simulink model "Cooperative_Quad_09_VelEst_02"  (R2017b)
settings: Solver=ode45  StartTime=0.0  StopTime=120  RelTol=1e-3  EnableMultiTasking=on
InitFcn:
  | Const_Vel_Est_02
values from neighbouring files (symbols this model uses):
  alpha = 1.0e-5    (= 1e-05)    [Cons_AMFC_Quad_New_01.m]    (also in Const_Vel_Est_02.m = 0.1; constant_Rev01_4Agents_10.m = 0.1; constant_Rev01_4Agents_9.m = 0.1)
  alpha_Slid = 0.01    [Cons_AMFC_Quad_New_01.m]    (also in Const_Vel_Est_02.m)
  AN = [     0 1 0 0 ... (first row only)    [Const_Vel_Est_02.m]    (also in constant_Rev01_4Agents_10.m; constant_Rev01_4Agents_9.m)
  B = 1e+0*eye(n)    [Cons_AMFC_Quad_New_01.m]    (also in Const_Vel_Est_02.m = 1e0*eye(n); constant_Rev01_4Agents_10.m = 1e0*eye(n); constant_Rev01_4Agents_9.m = 1e0*eye(n))
  BBT_inv = ((B'*B)^(-1))*B'    [Cons_AMFC_Quad_New_01.m]    (also in Const_Vel_Est_02.m; constant_Rev01_4Agents_10.m; constant_Rev01_4Agents_9.m)
  BN = [     1 0 0 0 ... (first row only)    [Const_Vel_Est_02.m]    (also in constant_Rev01_4Agents_10.m; constant_Rev01_4Agents_9.m)
  epsilon_struct = struct('data',epsilon_InitVal)    [Const_Vel_Est_02.m]    (also in constant_Rev01_4Agents_10.m; constant_Rev01_4Agents_9.m)
  g = 9.81    [Const_Vel_Est_02.m]    (also in Swing2d_01_const.m; constant_Rev01_4Agents_10.m; constant_Rev01_4Agents_9.m)
  gamma_0 = 1e-0*diag([1e-3*ones(3,1);1e-0*ones(3,1)])    [Cons_AMFC_Quad_New_01.m]    (also in Const_Vel_Est_02.m = 1e-1*diag([1e-3*ones(3,1);1e-0*ones(3,1)]); constant_Rev01_4Agents_10.m = 1e+1*diag([1e-3*ones(3,1);1e-0*ones(3,1)]); constant_Rev01_4Agents_9.m = 1e+1*diag([1e-3*ones(6,1);1e-0*ones(6,1)]))
  gamma_1 = 1e+2*diag([1e-3*ones(3,1);1e-0*ones(3,1)])    [Cons_AMFC_Quad_New_01.m]    (also in Const_Vel_Est_02.m; constant_Rev01_4Agents_10.m = 1e+3*diag([1e-3*ones(3,1);1e0*ones(3,1)]); constant_Rev01_4Agents_9.m = 1e+3*diag([1e-3*ones(6,1);1e0*ones(6,1)]))
  H = L + BN    [Const_Vel_Est_02.m]    (also in constant_Rev01_4Agents_10.m; constant_Rev01_4Agents_9.m)
  J = 1.2416e-3 * diag([1 1 2])    [Cons_AMFC_Quad_New_01.m]    (also in Const_Vel_Est_02.m = 1.2416e-3 * diag([1 1 2],0); constant_Rev01_4Agents_10.m = 1.2416e-3 * diag([1 1 2],0); constant_Rev01_4Agents_9.m = 1.2416e-3 * diag([1 1 2],0))
  k1 = 10    [Cons_AMFC_Quad_New_01.m]    (also in Const_Vel_Est_02.m = 1; constant_Rev01_4Agents_10.m = 1; constant_Rev01_4Agents_9.m = 1)
  k1o = 1000    [Cons_AMFC_Quad_New_01.m]    (also in Const_Vel_Est_02.m)
  k2 = 0.1    [Cons_AMFC_Quad_New_01.m]    (also in Const_Vel_Est_02.m; constant_Rev01_4Agents_10.m = 1; constant_Rev01_4Agents_9.m = 1)
  k2o = 100    [Cons_AMFC_Quad_New_01.m]    (also in Const_Vel_Est_02.m)
  Ka = 0.01    [Cons_AMFC_Quad_New_01.m]    (also in Const_Vel_Est_02.m; constant_Rev01_4Agents_10.m; constant_Rev01_4Agents_9.m)
  Kd = 0.01    [Cons_AMFC_Quad_New_01.m]    (also in Const_Vel_Est_02.m; constant_Rev01_4Agents_10.m; constant_Rev01_4Agents_9.m)
  Kf = 1.0e-5    (= 1e-05)    [Cons_AMFC_Quad_New_01.m]    (also in Const_Vel_Est_02.m; constant_Rev01_4Agents_10.m; constant_Rev01_4Agents_9.m)
  Kt = 0.0435 * Kf    (= 4.35e-07)    [Cons_AMFC_Quad_New_01.m]    (also in Const_Vel_Est_02.m = 1e-07; constant_Rev01_4Agents_10.m = 1e-07; constant_Rev01_4Agents_9.m = 1e-07)
  Lq = 0.2    [Const_Vel_Est_02.m]    (also in constant_Rev01_4Agents_10.m; constant_Rev01_4Agents_9.m)
  m = 6    [Cons_AMFC_Quad_New_01.m]    (also in Const_Vel_Est_02.m; Swing2d_01_const.m = 1)
  M = 2.95    [Cons_AMFC_Quad_New_01.m]    (also in Const_Vel_Est_02.m = 2; constant_Rev01_4Agents_10.m = 2; constant_Rev01_4Agents_9.m = 2)
  Mb_P = Mb_val_P*ones(np,1)    [Const_Vel_Est_02.m]
  Mb_V = Mb_val_V*ones(np,1)    [Const_Vel_Est_02.m]
  Mu_P = 10    [Const_Vel_Est_02.m]
  Mu_V = 10    [Const_Vel_Est_02.m]
  n = 6    [Cons_AMFC_Quad_New_01.m]    (also in Const_Vel_Est_02.m; constant_Rev01_4Agents_10.m; constant_Rev01_4Agents_9.m = 12)
  N = 4    [Const_Vel_Est_02.m]    (also in constant_Rev01_4Agents_10.m; constant_Rev01_4Agents_9.m)
  n0 = 3    [Const_Vel_Est_02.m]    (also in constant_Rev01_4Agents_10.m; constant_Rev01_4Agents_9.m)
  np = 2    [Const_Vel_Est_02.m]
  Observer_Gain = 100    [Const_Vel_Est_02.m]    (also in constant_Rev01_4Agents_10.m; constant_Rev01_4Agents_9.m)
  Observer_Gain1 = 100    [Const_Vel_Est_02.m]    (also in constant_Rev01_4Agents_10.m = 10; constant_Rev01_4Agents_9.m = 10)
  Q = 1e-1*eye(n)    [Cons_AMFC_Quad_New_01.m]    (also in Const_Vel_Est_02.m = 1e-2*eye(n); constant_Rev01_4Agents_10.m = 1e-3*eye(n); constant_Rev01_4Agents_9.m = 1e-3*eye(n))
  R = 1e+0*eye(m)    [Cons_AMFC_Quad_New_01.m]    (also in Const_Vel_Est_02.m = 1e-0*eye(n); constant_Rev01_4Agents_10.m = 1e-0*eye(n); constant_Rev01_4Agents_9.m = 1e-0*eye(n))
  rho_0 = 1e-1    (= 0.1)    [Cons_AMFC_Quad_New_01.m]    (also in Const_Vel_Est_02.m; constant_Rev01_4Agents_10.m = 10; constant_Rev01_4Agents_9.m = 10)
  rho_1 = 1e-0    (= 1)    [Cons_AMFC_Quad_New_01.m]    (also in Const_Vel_Est_02.m; constant_Rev01_4Agents_10.m = 0.1; constant_Rev01_4Agents_9.m = 0.1)
  T_struct = struct('data',T_InitVal)    [Const_Vel_Est_02.m]    (also in constant_Rev01_4Agents_10.m; constant_Rev01_4Agents_9.m)
  U_dot0_M = U_dot0_m*ones(n0,1)    [Const_Vel_Est_02.m]    (also in constant_Rev01_4Agents_10.m; constant_Rev01_4Agents_9.m)
  Upsilon_M = Upsilon_m*ones(n0,1)    [Const_Vel_Est_02.m]    (also in constant_Rev01_4Agents_10.m; constant_Rev01_4Agents_9.m)
undefined symbols (not defined in the file or in its folder): sigbuilder_block
(part 2 of 5)

== system Cooperative_Quad_09_VelEst_02/Agent #2/Relative estimations-2/Rel_21 ==
  A_local_XY : Inport
  P_local_XY : Inport  Port=2
  Differentiator1 : Subsystem
  Integrator1 : Integrator  InitialCondition=zeros(2,1)
  Integrator2 : Integrator  InitialCondition=zeros(2,1)
  Relative estimation1-2 : MATLAB Function  TreatAsAtomicUnit=on
  Relative estimation2 : MATLAB Function  TreatAsAtomicUnit=on
  Relative measurements2 : MATLAB Function  TreatAsAtomicUnit=on
  Sum : Sum  Inputs=|+-
  P_rel_21 : Outport
  V_rel_21 : Outport  Port=2
  wires:
  Sum/1 -> Relative estimation1-2/1(A_rel)
  [Acc1_XY] -> Sum/2
  [Pos1_XY] -> Relative measurements2/1(P_other)
  Differentiator1/1(Dx_d) -> Relative estimation1-2/2(dv)
  Relative estimation1-2/1(DV_est) -> Integrator1/1
  Relative estimation2/1(DP_est) -> Integrator2/1
  P_local_XY/1 -> Relative measurements2/2(P_local)
  A_local_XY/1 -> Sum/1
  Integrator1/1 -> Relative estimation2/1(V_rel), V_rel_21/1, Relative estimation1-2/3(V_est)
  Relative measurements2/1(d) -> Relative estimation2/2(dp), Differentiator1/1(x_d)
  Integrator2/1 -> Relative estimation2/3(P_est), P_rel_21/1

== system Cooperative_Quad_09_VelEst_02/Agent #2/Relative estimations-2/Rel_23 ==
  A_local_XY : Inport
  P_local_XY : Inport  Port=2
  Differentiator1 : Subsystem
  Integrator1 : Integrator  InitialCondition=zeros(2,1)
  Integrator2 : Integrator  InitialCondition=zeros(2,1)
  Relative estimation1-2 : MATLAB Function  TreatAsAtomicUnit=on
  Relative estimation2 : MATLAB Function  TreatAsAtomicUnit=on
  Relative measurements2 : MATLAB Function  TreatAsAtomicUnit=on
  Sum : Sum  Inputs=|+-
  P_rel_23 : Outport
  V_rel_23 : Outport  Port=2
  wires:
  Integrator2/1 -> P_rel_23/1, Relative estimation2/3(P_est)
  Relative measurements2/1(d) -> Differentiator1/1(x_d), Relative estimation2/2(dp)
  Integrator1/1 -> V_rel_23/1, Relative estimation2/1(V_rel), Relative estimation1-2/3(V_est)
  A_local_XY/1 -> Sum/1
  P_local_XY/1 -> Relative measurements2/2(P_local)
  Relative estimation2/1(DP_est) -> Integrator2/1
  Relative estimation1-2/1(DV_est) -> Integrator1/1
  Differentiator1/1(Dx_d) -> Relative estimation1-2/2(dv)
  [Pos3_XY] -> Relative measurements2/1(P_other)
  [Acc3_XY] -> Sum/2
  Sum/1 -> Relative estimation1-2/1(A_rel)

== system Cooperative_Quad_09_VelEst_02/Agent #2/Relative estimations-2/Rel_24 ==
  A_local_XY : Inport
  P_local_XY : Inport  Port=2
  Differentiator1 : Subsystem
  Integrator1 : Integrator  InitialCondition=zeros(2,1)
  Integrator2 : Integrator  InitialCondition=zeros(2,1)
  Relative estimation1 : MATLAB Function  TreatAsAtomicUnit=on
  Relative estimation2 : MATLAB Function  TreatAsAtomicUnit=on
  Relative measurements1 : MATLAB Function  TreatAsAtomicUnit=on
  Sum : Sum  Inputs=|+-
  P_rel_24 : Outport
  V_rel_24 : Outport  Port=2
  wires:
  Sum/1 -> Relative estimation2/1(A_rel)
  [Acc4_XY] -> Sum/2
  [Pos4_XY] -> Relative measurements1/1(P_other)
  Differentiator1/1(Dx_d) -> Relative estimation2/2(dv)
  Relative estimation2/1(DV_est) -> Integrator1/1
  Relative estimation1/1(DP_est) -> Integrator2/1
  P_local_XY/1 -> Relative measurements1/2(P_local)
  A_local_XY/1 -> Sum/1
  Integrator1/1 -> Relative estimation1/1(V_rel), V_rel_24/1, Relative estimation2/3(V_est)
  Relative measurements1/1(d) -> Relative estimation1/2(dp), Differentiator1/1(x_d)
  Integrator2/1 -> Relative estimation1/3(P_est), P_rel_24/1

== system Cooperative_Quad_09_VelEst_02/Agent #3/Decenteralized Cooperaive Controller #3/Ali-3 ==
  x : Inport
  xd : Inport  Port=2
  Controller interpreter-3 : MATLAB Function  TreatAsAtomicUnit=on
  Controller interpreter1-3 : MATLAB Function  TreatAsAtomicUnit=on
  Rotational-3 : Subsystem
  Translational-3 : Subsystem
  u : Outport
  wires:
  Controller interpreter-3/2(PHI_d) -> Rotational-3/1(x_rd)
  Rotational-3/1(ur) -> Controller interpreter1-3/2(ur)
  Controller interpreter1-3/1(u) -> u/1
  Controller interpreter-3/1(u0) -> Controller interpreter1-3/1(u0t)
  xd/1 -> Translational-3/1(x_td)
  x/1 -> Rotational-3/2(X), Translational-3/2(x_t)
  Translational-3/1(ut) -> Controller interpreter-3/1(u)

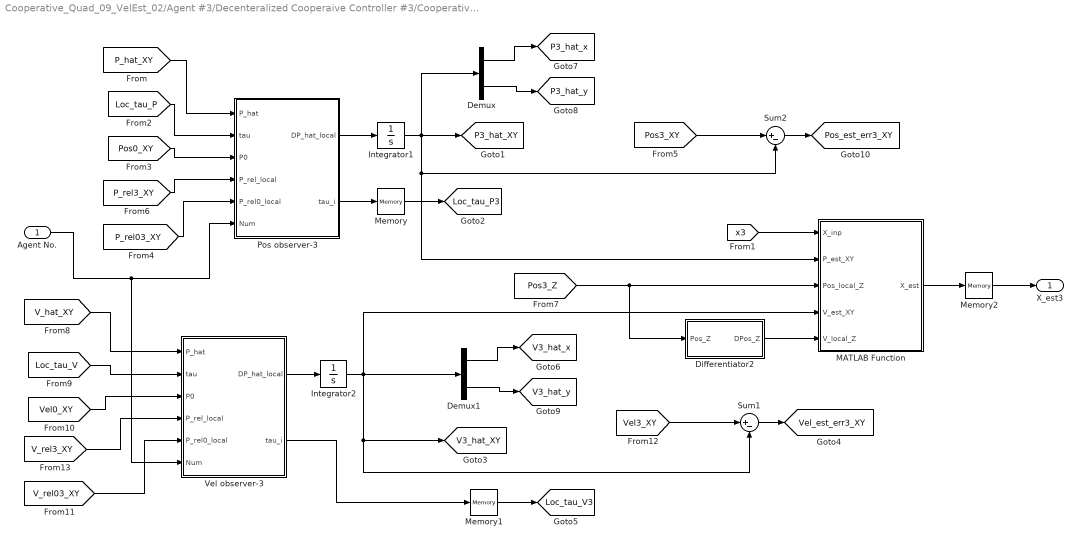
== system Cooperative_Quad_09_VelEst_02/Agent #3/Decenteralized Cooperaive Controller #3/Cooperative Observers for X-3 ==
  Agent No. : Inport
  Demux : Demux  Outputs=2
  Demux1 : Demux  Outputs=2
  Differentiator2 : Subsystem
  Integrator1 : Integrator  InitialCondition=zeros(np,1)
  Integrator2 : Integrator  InitialCondition=zeros(np,1)
  MATLAB Function : MATLAB Function  TreatAsAtomicUnit=on
  Memory : Memory  InitialCondition=zeros(np,1)
  Memory1 : Memory  InitialCondition=zeros(np,1)
  Memory2 : Memory  InitialCondition=zeros(2*n,1)
  Pos observer-3 : MATLAB Function  TreatAsAtomicUnit=on
  Sum1 : Sum  Inputs=|+-
  Sum2 : Sum  Inputs=|+-
  Vel observer-3 : MATLAB Function  TreatAsAtomicUnit=on
  X_est3 : Outport
  tag scope: Loc_tau_P3=global, Loc_tau_V3=global, P3_hat_XY=global, P3_hat_x=global, P3_hat_y=global, Pos_est_err3_XY=global, V3_hat_XY=global, V3_hat_x=global, V3_hat_y=global, Vel_est_err3_XY=global
  wires:
  [Pos3_XY] -> Sum2/1
  [Loc_tau_P] -> Pos observer-3/2(tau)
  [P_rel03_XY] -> Pos observer-3/5(P_rel0_local)
  Pos observer-3/1(DP_hat_local) -> Integrator1/1
  Pos observer-3/2(tau_i) -> Memory/1
  Demux/1 -> [P3_hat_x]
  Memory/1 -> [Loc_tau_P3]
  [Pos0_XY] -> Pos observer-3/3(P0)
  [P_hat_XY] -> Pos observer-3/1(P_hat)
  Sum2/1 -> [Pos_est_err3_XY]
  [P_rel3_XY] -> Pos observer-3/4(P_rel_local)
  Demux/2 -> [P3_hat_y]
  Integrator1/1 -> Sum2/2, MATLAB Function/2(P_est_XY), Demux/1, [P3_hat_XY]
  Agent No./1 -> Vel observer-3/6(Num), Pos observer-3/6(Num)
  MATLAB Function/1(X_est) -> Memory2/1
  [x3] -> MATLAB Function/1(X_inp)
  [Pos3_Z] -> Differentiator2/1(Pos_Z), MATLAB Function/3(Pos_local_Z)
  Differentiator2/1(DPos_Z) -> MATLAB Function/5(V_local_Z)
  [Vel3_XY] -> Sum1/1
  Integrator2/1 -> Sum1/2, [V3_hat_XY], Demux1/1, MATLAB Function/4(V_est_XY)
  Demux1/2 -> [V3_hat_y]
  [V_rel3_XY] -> Vel observer-3/4(P_rel_local)
  [Loc_tau_V] -> Vel observer-3/2(tau)
  [V_hat_XY] -> Vel observer-3/1(P_hat)
  Sum1/1 -> [Vel_est_err3_XY]
  [V_rel03_XY] -> Vel observer-3/5(P_rel0_local)
  [Vel0_XY] -> Vel observer-3/3(P0)
  Demux1/1 -> [V3_hat_x]
  Memory1/1 -> [Loc_tau_V3]
  Vel observer-3/2(tau_i) -> Memory1/1
  Vel observer-3/1(DP_hat_local) -> Integrator2/1
  Memory2/1 -> X_est3/1

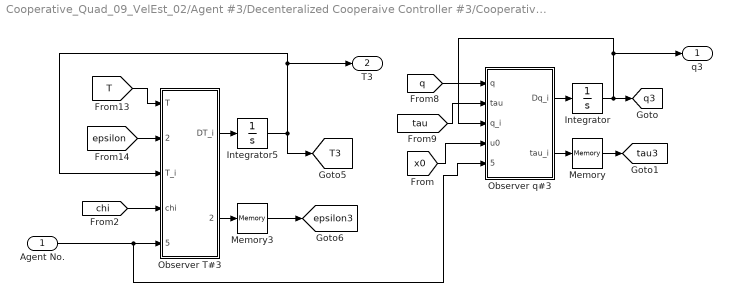
== system Cooperative_Quad_09_VelEst_02/Agent #3/Decenteralized Cooperaive Controller #3/Cooperative Observers for Xd-3 ==
  Agent No. : Inport
  Integrator : Integrator  InitialCondition=zeros(n0,1)
  Integrator5 : Integrator  InitialCondition=zeros(N+1,n0)
  Memory : Memory  InitialCondition=zeros(n0,1)
  Memory3 : Memory  InitialCondition=zeros(N+1,n0)
  Observer T#3 : MATLAB Function  TreatAsAtomicUnit=on
  Observer q#3 : MATLAB Function  TreatAsAtomicUnit=on
  q3 : Outport
  T3 : Outport  Port=2
  tag scope: T3=global, epsilon3=global, q3=global, tau3=global
  wires:
  [chi] -> Observer T#3/4(chi)
  [epsilon] -> Observer T#3/2(epsilon)
  Observer T#3/1(DT_i) -> Integrator5/1
  [T] -> Observer T#3/1(T)
  Observer T#3/2(epsilon_i) -> Memory3/1
  Observer q#3/1(Dq_i) -> Integrator/1
  Memory/1 -> [tau3]
  [x0] -> Observer q#3/4(u0)
  Observer q#3/2(tau_i) -> Memory/1
  Agent No./1 -> Observer q#3/5(Agent_Num), Observer T#3/5(Agent_Num)
  Integrator5/1 -> [T3], T3/1, Observer T#3/3(T_i)
  [q] -> Observer q#3/1(q)
  Integrator/1 -> [q3], q3/1, Observer q#3/3(q_i)
  [tau] -> Observer q#3/2(tau)
  Memory3/1 -> [epsilon3]

== system Cooperative_Quad_09_VelEst_02/Agent #3/Decenteralized Cooperaive Controller #3/Subsystem ==
  In1 : Inport
  Demux : Demux  Outputs=3
  Mux : Mux  Inputs=3
  Transport Delay1 : TransportDelay  DelayTime=5
  Transport Delay2 : TransportDelay  DelayTime=5
  Out1 : Outport
  wires:
  In1/1 -> Demux/1
  Demux/1 -> Transport Delay1/1
  Demux/2 -> Transport Delay2/1
  Mux/1 -> Out1/1
  Transport Delay2/1 -> Mux/2
  Transport Delay1/1 -> Mux/1
  Demux/3 -> Mux/3

== system Cooperative_Quad_09_VelEst_02/Agent #3/Relative estimations-3/Rel_30 ==
  A_local_XY : Inport
  P_local_XY : Inport  Port=2
  Differentiator1 : Subsystem
  Integrator1 : Integrator  InitialCondition=zeros(2,1)
  Integrator2 : Integrator  InitialCondition=zeros(2,1)
  Relative estimation1 : MATLAB Function  TreatAsAtomicUnit=on
  Relative estimation2 : MATLAB Function  TreatAsAtomicUnit=on
  Relative measurements1 : MATLAB Function  TreatAsAtomicUnit=on
  Sum : Sum  Inputs=|+-
  P_rel_30 : Outport
  V_rel_30 : Outport  Port=2
  wires:
  Sum/1 -> Relative estimation2/1(A_rel)
  [Acc0_XY] -> Sum/2
  [Pos0_XY] -> Relative measurements1/1(P_other)
  Differentiator1/1(Dx_d) -> Relative estimation2/2(dv)
  Relative estimation2/1(DV_est) -> Integrator1/1
  Relative estimation1/1(DP_est) -> Integrator2/1
  P_local_XY/1 -> Relative measurements1/2(P_local)
  A_local_XY/1 -> Sum/1
  Integrator1/1 -> Relative estimation1/1(V_rel), V_rel_30/1, Relative estimation2/3(V_est)
  Relative measurements1/1(d) -> Relative estimation1/2(dp), Differentiator1/1(x_d)
  Integrator2/1 -> Relative estimation1/3(P_est), P_rel_30/1

== system Cooperative_Quad_09_VelEst_02/Agent #3/Relative estimations-3/Rel_31 ==
  A_local_XY : Inport
  P_local_XY : Inport  Port=2
  Differentiator1 : Subsystem
  Integrator1 : Integrator  InitialCondition=zeros(2,1)
  Integrator2 : Integrator  InitialCondition=zeros(2,1)
  Relative estimation1-2 : MATLAB Function  TreatAsAtomicUnit=on
  Relative estimation2 : MATLAB Function  TreatAsAtomicUnit=on
  Relative measurements2 : MATLAB Function  TreatAsAtomicUnit=on
  Sum : Sum  Inputs=|+-
  P_rel_31 : Outport
  V_rel_31 : Outport  Port=2
  wires:
  Integrator2/1 -> P_rel_31/1, Relative estimation2/3(P_est)
  Relative measurements2/1(d) -> Differentiator1/1(x_d), Relative estimation2/2(dp)
  Integrator1/1 -> Relative estimation1-2/3(V_est), V_rel_31/1, Relative estimation2/1(V_rel)
  A_local_XY/1 -> Sum/1
  P_local_XY/1 -> Relative measurements2/2(P_local)
  Relative estimation2/1(DP_est) -> Integrator2/1
  Relative estimation1-2/1(DV_est) -> Integrator1/1
  Differentiator1/1(Dx_d) -> Relative estimation1-2/2(dv)
  [Pos1_XY] -> Relative measurements2/1(P_other)
  [Acc1_XY] -> Sum/2
  Sum/1 -> Relative estimation1-2/1(A_rel)

== system Cooperative_Quad_09_VelEst_02/Agent #3/Relative estimations-3/Rel_32 ==
  A_local_XY : Inport
  P_local_XY : Inport  Port=2
  Differentiator1 : Subsystem
  Integrator1 : Integrator  InitialCondition=zeros(2,1)
  Integrator2 : Integrator  InitialCondition=zeros(2,1)
  Relative estimation1-2 : MATLAB Function  TreatAsAtomicUnit=on
  Relative estimation2 : MATLAB Function  TreatAsAtomicUnit=on
  Relative measurements2 : MATLAB Function  TreatAsAtomicUnit=on
  Sum : Sum  Inputs=|+-
  P_rel_32 : Outport
  V_rel_32 : Outport  Port=2
  wires:
  Sum/1 -> Relative estimation1-2/1(A_rel)
  [Acc2_XY] -> Sum/2
  [Pos2_XY] -> Relative measurements2/1(P_other)
  Differentiator1/1(Dx_d) -> Relative estimation1-2/2(dv)
  Relative estimation1-2/1(DV_est) -> Integrator1/1
  Relative estimation2/1(DP_est) -> Integrator2/1
  P_local_XY/1 -> Relative measurements2/2(P_local)
  A_local_XY/1 -> Sum/1
  Integrator1/1 -> Relative estimation1-2/3(V_est), Relative estimation2/1(V_rel), V_rel_32/1
  Relative measurements2/1(d) -> Relative estimation2/2(dp), Differentiator1/1(x_d)
  Integrator2/1 -> Relative estimation2/3(P_est), P_rel_32/1

== system Cooperative_Quad_09_VelEst_02/Agent #3/Relative estimations-3/Rel_34 ==
  A_local_XY : Inport
  P_local_XY : Inport  Port=2
  Differentiator1 : Subsystem
  Integrator1 : Integrator  InitialCondition=zeros(2,1)
  Integrator2 : Integrator  InitialCondition=zeros(2,1)
  Relative estimation1 : MATLAB Function  TreatAsAtomicUnit=on
  Relative estimation2 : MATLAB Function  TreatAsAtomicUnit=on
  Relative measurements1 : MATLAB Function  TreatAsAtomicUnit=on
  Sum : Sum  Inputs=|+-
  P_rel_34 : Outport
  V_rel_34 : Outport  Port=2
  wires:
  Integrator2/1 -> P_rel_34/1, Relative estimation1/3(P_est)
  Relative measurements1/1(d) -> Differentiator1/1(x_d), Relative estimation1/2(dp)
  Integrator1/1 -> Relative estimation2/3(V_est), V_rel_34/1, Relative estimation1/1(V_rel)
  A_local_XY/1 -> Sum/1
  P_local_XY/1 -> Relative measurements1/2(P_local)
  Relative estimation1/1(DP_est) -> Integrator2/1
  Relative estimation2/1(DV_est) -> Integrator1/1
  Differentiator1/1(Dx_d) -> Relative estimation2/2(dv)
  [Pos4_XY] -> Relative measurements1/1(P_other)
  [Acc4_XY] -> Sum/2
  Sum/1 -> Relative estimation2/1(A_rel)

== system Cooperative_Quad_09_VelEst_02/Agent #4/Decenteralized Cooperaive Controller #4/Ali-4 ==
  x : Inport
  xd : Inport  Port=2
  Controller interpreter-4 : MATLAB Function  TreatAsAtomicUnit=on
  Controller interpreter1-4 : MATLAB Function  TreatAsAtomicUnit=on
  Rotational-4 : Subsystem
  Translational-4 : Subsystem
  u : Outport
  wires:
  Translational-4/1(ut) -> Controller interpreter-4/1(u)
  x/1 -> Translational-4/2(x_t), Rotational-4/2(X)
  xd/1 -> Translational-4/1(x_td)
  Controller interpreter-4/1(u0) -> Controller interpreter1-4/1(u0t)
  Controller interpreter1-4/1(u) -> u/1
  Rotational-4/1(ur) -> Controller interpreter1-4/2(ur)
  Controller interpreter-4/2(PHI_d) -> Rotational-4/1(x_rd)

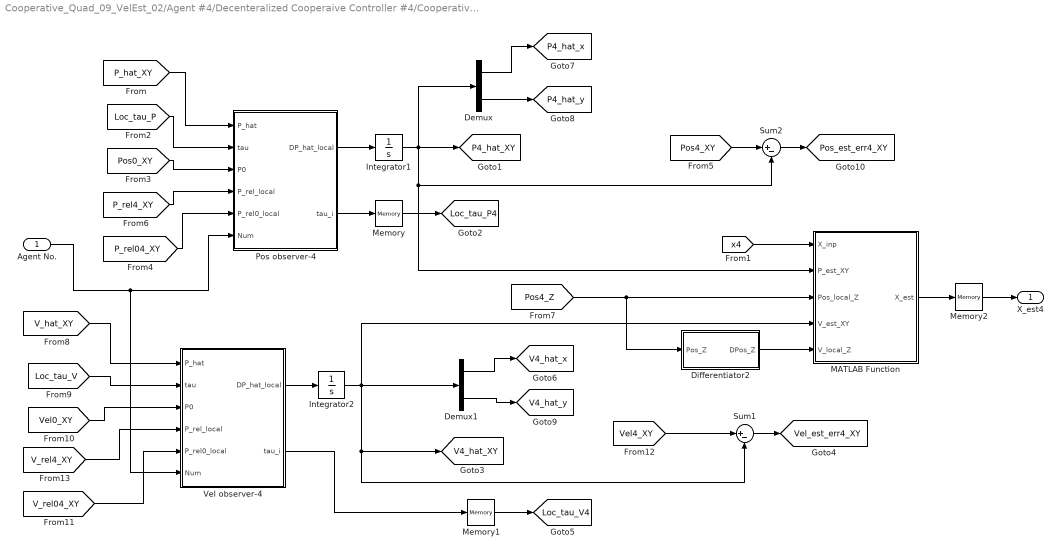
== system Cooperative_Quad_09_VelEst_02/Agent #4/Decenteralized Cooperaive Controller #4/Cooperative Observers for X-4 ==
  Agent No. : Inport
  Demux : Demux  Outputs=2
  Demux1 : Demux  Outputs=2
  Differentiator2 : Subsystem
  Integrator1 : Integrator  InitialCondition=zeros(np,1)
  Integrator2 : Integrator  InitialCondition=zeros(np,1)
  MATLAB Function : MATLAB Function  TreatAsAtomicUnit=on
  Memory : Memory  InitialCondition=zeros(np,1)
  Memory1 : Memory  InitialCondition=zeros(np,1)
  Memory2 : Memory  InitialCondition=zeros(2*n,1)
  Pos observer-4 : MATLAB Function  TreatAsAtomicUnit=on
  Sum1 : Sum  Inputs=|+-
  Sum2 : Sum  Inputs=|+-
  Vel observer-4 : MATLAB Function  TreatAsAtomicUnit=on
  X_est4 : Outport
  tag scope: Loc_tau_P4=global, Loc_tau_V4=global, P4_hat_XY=global, P4_hat_x=global, P4_hat_y=global, Pos_est_err4_XY=global, V4_hat_XY=global, V4_hat_x=global, V4_hat_y=global, Vel_est_err4_XY=global
  wires:
  Vel observer-4/1(DP_hat_local) -> Integrator2/1
  Vel observer-4/2(tau_i) -> Memory1/1
  Memory1/1 -> [Loc_tau_V4]
  Demux1/1 -> [V4_hat_x]
  [Vel0_XY] -> Vel observer-4/3(P0)
  [V_rel04_XY] -> Vel observer-4/5(P_rel0_local)
  Sum1/1 -> [Vel_est_err4_XY]
  [V_hat_XY] -> Vel observer-4/1(P_hat)
  [Loc_tau_V] -> Vel observer-4/2(tau)
  [V_rel4_XY] -> Vel observer-4/4(P_rel_local)
  Demux1/2 -> [V4_hat_y]
  Integrator2/1 -> MATLAB Function/4(V_est_XY), Demux1/1, [V4_hat_XY], Sum1/2
  [Vel4_XY] -> Sum1/1
  Differentiator2/1(DPos_Z) -> MATLAB Function/5(V_local_Z)
  [Pos4_Z] -> MATLAB Function/3(Pos_local_Z), Differentiator2/1(Pos_Z)
  [x4] -> MATLAB Function/1(X_inp)
  MATLAB Function/1(X_est) -> Memory2/1
  Agent No./1 -> Pos observer-4/6(Num), Vel observer-4/6(Num)
  Integrator1/1 -> [P4_hat_XY], Demux/1, MATLAB Function/2(P_est_XY), Sum2/2
  Demux/2 -> [P4_hat_y]
  [P_rel4_XY] -> Pos observer-4/4(P_rel_local)
  Sum2/1 -> [Pos_est_err4_XY]
  [P_hat_XY] -> Pos observer-4/1(P_hat)
  [Pos0_XY] -> Pos observer-4/3(P0)
  Memory/1 -> [Loc_tau_P4]
  Demux/1 -> [P4_hat_x]
  Pos observer-4/2(tau_i) -> Memory/1
  Pos observer-4/1(DP_hat_local) -> Integrator1/1
  [P_rel04_XY] -> Pos observer-4/5(P_rel0_local)
  [Loc_tau_P] -> Pos observer-4/2(tau)
  [Pos4_XY] -> Sum2/1
  Memory2/1 -> X_est4/1

== system Cooperative_Quad_09_VelEst_02/Agent #4/Decenteralized Cooperaive Controller #4/Cooperative Observers for Xd-4 ==
  Agent No. : Inport
  Integrator : Integrator  InitialCondition=zeros(n0,1)
  Integrator5 : Integrator  InitialCondition=zeros(N+1,n0)
  Memory : Memory  InitialCondition=zeros(n0,1)
  Memory3 : Memory  InitialCondition=zeros(N+1,n0)
  Observer T#4 : MATLAB Function  TreatAsAtomicUnit=on
  Observer q#4 : MATLAB Function  TreatAsAtomicUnit=on
  q4 : Outport
  T4 : Outport  Port=2
  tag scope: T4=global, epsilon4=global, q4=global, tau4=global
  wires:
  Memory3/1 -> [epsilon4]
  [tau] -> Observer q#4/2(tau)
  Integrator/1 -> Observer q#4/3(q_i), q4/1, [q4]
  [q] -> Observer q#4/1(q)
  Integrator5/1 -> Observer T#4/3(T_i), T4/1, [T4]
  Agent No./1 -> Observer T#4/5(Agent_Num), Observer q#4/5(Agent_Num)
  Observer q#4/2(tau_i) -> Memory/1
  [x0] -> Observer q#4/4(u0)
  Memory/1 -> [tau4]
  Observer q#4/1(Dq_i) -> Integrator/1
  Observer T#4/2(epsilon_i) -> Memory3/1
  [T] -> Observer T#4/1(T)
  Observer T#4/1(DT_i) -> Integrator5/1
  [epsilon] -> Observer T#4/2(epsilon)
  [chi] -> Observer T#4/4(chi)

== system Cooperative_Quad_09_VelEst_02/Agent #4/Decenteralized Cooperaive Controller #4/Subsystem ==
  In1 : Inport
  Demux : Demux  Outputs=3
  Mux : Mux  Inputs=3
  Transport Delay1 : TransportDelay  DelayTime=5
  Transport Delay2 : TransportDelay  DelayTime=5
  Out1 : Outport
  wires:
  Demux/3 -> Mux/3
  Transport Delay1/1 -> Mux/1
  Transport Delay2/1 -> Mux/2
  Mux/1 -> Out1/1
  Demux/2 -> Transport Delay2/1
  Demux/1 -> Transport Delay1/1
  In1/1 -> Demux/1

== system Cooperative_Quad_09_VelEst_02/Agent #4/Relative estimations-4/Rel_40 ==
  A_local_XY : Inport
  P_local_XY : Inport  Port=2
  Differentiator1 : Subsystem
  Integrator1 : Integrator  InitialCondition=zeros(2,1)
  Integrator2 : Integrator  InitialCondition=zeros(2,1)
  Relative estimation1 : MATLAB Function  TreatAsAtomicUnit=on
  Relative estimation2 : MATLAB Function  TreatAsAtomicUnit=on
  Relative measurements1 : MATLAB Function  TreatAsAtomicUnit=on
  Sum : Sum  Inputs=|+-
  P_rel_40 : Outport
  V_rel_40 : Outport  Port=2
  wires:
  Integrator2/1 -> P_rel_40/1, Relative estimation1/3(P_est)
  Relative measurements1/1(d) -> Differentiator1/1(x_d), Relative estimation1/2(dp)
  Integrator1/1 -> Relative estimation2/3(V_est), V_rel_40/1, Relative estimation1/1(V_rel)
  A_local_XY/1 -> Sum/1
  P_local_XY/1 -> Relative measurements1/2(P_local)
  Relative estimation1/1(DP_est) -> Integrator2/1
  Relative estimation2/1(DV_est) -> Integrator1/1
  Differentiator1/1(Dx_d) -> Relative estimation2/2(dv)
  [Pos0_XY] -> Relative measurements1/1(P_other)
  [Acc0_XY] -> Sum/2
  Sum/1 -> Relative estimation2/1(A_rel)

== system Cooperative_Quad_09_VelEst_02/Agent #4/Relative estimations-4/Rel_41 ==
  A_local_XY : Inport
  P_local_XY : Inport  Port=2
  Differentiator1 : Subsystem
  Integrator1 : Integrator  InitialCondition=zeros(2,1)
  Integrator2 : Integrator  InitialCondition=zeros(2,1)
  Relative estimation1-2 : MATLAB Function  TreatAsAtomicUnit=on
  Relative estimation2 : MATLAB Function  TreatAsAtomicUnit=on
  Relative measurements2 : MATLAB Function  TreatAsAtomicUnit=on
  Sum : Sum  Inputs=|+-
  P_rel_41 : Outport
  V_rel_41 : Outport  Port=2
  wires:
  Sum/1 -> Relative estimation1-2/1(A_rel)
  [Acc1_XY] -> Sum/2
  [Pos1_XY] -> Relative measurements2/1(P_other)
  Differentiator1/1(Dx_d) -> Relative estimation1-2/2(dv)
  Relative estimation1-2/1(DV_est) -> Integrator1/1
  Relative estimation2/1(DP_est) -> Integrator2/1
  P_local_XY/1 -> Relative measurements2/2(P_local)
  A_local_XY/1 -> Sum/1
  Integrator1/1 -> Relative estimation2/1(V_rel), V_rel_41/1, Relative estimation1-2/3(V_est)
  Relative measurements2/1(d) -> Relative estimation2/2(dp), Differentiator1/1(x_d)
  Integrator2/1 -> Relative estimation2/3(P_est), P_rel_41/1

== system Cooperative_Quad_09_VelEst_02/Agent #4/Relative estimations-4/Rel_42 ==
  A_local_XY : Inport
  P_local_XY : Inport  Port=2
  Differentiator1 : Subsystem
  Integrator1 : Integrator  InitialCondition=zeros(2,1)
  Integrator2 : Integrator  InitialCondition=zeros(2,1)
  Relative estimation1-2 : MATLAB Function  TreatAsAtomicUnit=on
  Relative estimation2 : MATLAB Function  TreatAsAtomicUnit=on
  Relative measurements2 : MATLAB Function  TreatAsAtomicUnit=on
  Sum : Sum  Inputs=|+-
  P_rel_42 : Outport
  V_rel_42 : Outport  Port=2
  wires:
  Integrator2/1 -> P_rel_42/1, Relative estimation2/3(P_est)
  Relative measurements2/1(d) -> Differentiator1/1(x_d), Relative estimation2/2(dp)
  Integrator1/1 -> V_rel_42/1, Relative estimation2/1(V_rel), Relative estimation1-2/3(V_est)
  A_local_XY/1 -> Sum/1
  P_local_XY/1 -> Relative measurements2/2(P_local)
  Relative estimation2/1(DP_est) -> Integrator2/1
  Relative estimation1-2/1(DV_est) -> Integrator1/1
  Differentiator1/1(Dx_d) -> Relative estimation1-2/2(dv)
  [Pos2_XY] -> Relative measurements2/1(P_other)
  [Acc2_XY] -> Sum/2
  Sum/1 -> Relative estimation1-2/1(A_rel)

== system Cooperative_Quad_09_VelEst_02/Agent #4/Relative estimations-4/Rel_43 ==
  A_local_XY : Inport
  P_local_XY : Inport  Port=2
  Differentiator1 : Subsystem
  Integrator1 : Integrator  InitialCondition=zeros(2,1)
  Integrator2 : Integrator  InitialCondition=zeros(2,1)
  Relative estimation1 : MATLAB Function  TreatAsAtomicUnit=on
  Relative estimation2 : MATLAB Function  TreatAsAtomicUnit=on
  Relative measurements1 : MATLAB Function  TreatAsAtomicUnit=on
  Sum : Sum  Inputs=|+-
  P_rel_43 : Outport
  V_rel_43 : Outport  Port=2
  wires:
  Sum/1 -> Relative estimation2/1(A_rel)
  [Acc3_XY] -> Sum/2
  [Pos3_XY] -> Relative measurements1/1(P_other)
  Differentiator1/1(Dx_d) -> Relative estimation2/2(dv)
  Relative estimation2/1(DV_est) -> Integrator1/1
  Relative estimation1/1(DP_est) -> Integrator2/1
  P_local_XY/1 -> Relative measurements1/2(P_local)
  A_local_XY/1 -> Sum/1
  Integrator1/1 -> Relative estimation1/1(V_rel), V_rel_43/1, Relative estimation2/3(V_est)
  Relative measurements1/1(d) -> Relative estimation1/2(dp), Differentiator1/1(x_d)
  Integrator2/1 -> Relative estimation1/3(P_est), P_rel_43/1

== system Cooperative_Quad_09_VelEst_02/Data Bus /Communications for controllers/For matrix Plot ==
  P : Inport
  MATLAB Function : MATLAB Function  TreatAsAtomicUnit=on
  Scope24 : Scope
  To Workspace : ToWorkspace  VariableName=P1_T  SaveFormat=Structure With Time  SampleTime=-1
  wires:
  P/1 -> MATLAB Function/1(u)
  MATLAB Function/1(y) -> Scope24/1, To Workspace/1

== system Cooperative_Quad_09_VelEst_02/Data Bus /Communications for controllers/For matrix Plot1 ==
  P : Inport
  MATLAB Function : MATLAB Function  TreatAsAtomicUnit=on
  Scope24 : Scope
  To Workspace : ToWorkspace  VariableName=P2_T  SaveFormat=Structure With Time  SampleTime=-1
  wires:
  MATLAB Function/1(y) -> Scope24/1, To Workspace/1
  P/1 -> MATLAB Function/1(u)

== system Cooperative_Quad_09_VelEst_02/Data Bus /Communications for controllers/For matrix Plot16 ==
  P : Inport
  MATLAB Function : MATLAB Function  TreatAsAtomicUnit=on
  Scope24 : Scope
  To Workspace : ToWorkspace  VariableName=P1_R  SaveFormat=Structure With Time  SampleTime=-1
  wires:
  MATLAB Function/1(y) -> To Workspace/1, Scope24/1
  P/1 -> MATLAB Function/1(u)

== system Cooperative_Quad_09_VelEst_02/Data Bus /Communications for controllers/For matrix Plot17 ==
  P : Inport
  MATLAB Function : MATLAB Function  TreatAsAtomicUnit=on
  Scope24 : Scope
  To Workspace : ToWorkspace  VariableName=P2_R  SaveFormat=Structure With Time  SampleTime=-1
  wires:
  P/1 -> MATLAB Function/1(u)
  MATLAB Function/1(y) -> To Workspace/1, Scope24/1

== system Cooperative_Quad_09_VelEst_02/Data Bus /Communications for controllers/For matrix Plot18 ==
  P : Inport
  MATLAB Function : MATLAB Function  TreatAsAtomicUnit=on
  Scope24 : Scope
  To Workspace : ToWorkspace  VariableName=P3_R  SaveFormat=Structure With Time  SampleTime=-1
  wires:
  P/1 -> MATLAB Function/1(u)
  MATLAB Function/1(y) -> To Workspace/1, Scope24/1

== system Cooperative_Quad_09_VelEst_02/Data Bus /Communications for controllers/For matrix Plot19 ==
  P : Inport
  MATLAB Function : MATLAB Function  TreatAsAtomicUnit=on
  Scope24 : Scope
  To Workspace : ToWorkspace  VariableName=P4_R  SaveFormat=Structure With Time  SampleTime=-1
  wires:
  MATLAB Function/1(y) -> To Workspace/1, Scope24/1
  P/1 -> MATLAB Function/1(u)

== system Cooperative_Quad_09_VelEst_02/Data Bus /Communications for controllers/For matrix Plot2 ==
  P : Inport
  MATLAB Function : MATLAB Function  TreatAsAtomicUnit=on
  Scope24 : Scope
  To Workspace : ToWorkspace  VariableName=P3_T  SaveFormat=Structure With Time  SampleTime=-1
  wires:
  MATLAB Function/1(y) -> Scope24/1, To Workspace/1
  P/1 -> MATLAB Function/1(u)

== system Cooperative_Quad_09_VelEst_02/Data Bus /Communications for controllers/For matrix Plot20 ==
  A_hat : Inport
  MATLAB Function : MATLAB Function  TreatAsAtomicUnit=on
  Scope24 : Scope
  To Workspace : ToWorkspace  VariableName=A_hat1_R  SaveFormat=Structure With Time  SampleTime=-1
  wires:
  A_hat/1 -> MATLAB Function/1(u)
  MATLAB Function/1(y) -> To Workspace/1, Scope24/1

== system Cooperative_Quad_09_VelEst_02/Data Bus /Communications for controllers/For matrix Plot21 ==
  A_hat : Inport
  MATLAB Function : MATLAB Function  TreatAsAtomicUnit=on
  Scope24 : Scope
  To Workspace : ToWorkspace  VariableName=A_hat2_R  SaveFormat=Structure With Time  SampleTime=-1
  wires:
  MATLAB Function/1(y) -> To Workspace/1, Scope24/1
  A_hat/1 -> MATLAB Function/1(u)

== system Cooperative_Quad_09_VelEst_02/Data Bus /Communications for controllers/For matrix Plot22 ==
  A_hat : Inport
  MATLAB Function : MATLAB Function  TreatAsAtomicUnit=on
  Scope24 : Scope
  To Workspace : ToWorkspace  VariableName=A_hat3_R  SaveFormat=Structure With Time  SampleTime=-1
  wires:
  A_hat/1 -> MATLAB Function/1(u)
  MATLAB Function/1(y) -> To Workspace/1, Scope24/1

== system Cooperative_Quad_09_VelEst_02/Data Bus /Communications for controllers/For matrix Plot23 ==
  A_hat : Inport
  MATLAB Function : MATLAB Function  TreatAsAtomicUnit=on
  Scope24 : Scope
  To Workspace : ToWorkspace  VariableName=A_hat4_R  SaveFormat=Structure With Time  SampleTime=-1
  wires:
  MATLAB Function/1(y) -> To Workspace/1, Scope24/1
  A_hat/1 -> MATLAB Function/1(u)

== system Cooperative_Quad_09_VelEst_02/Data Bus /Communications for controllers/For matrix Plot3 ==
  P : Inport
  MATLAB Function : MATLAB Function  TreatAsAtomicUnit=on
  Scope24 : Scope
  To Workspace : ToWorkspace  VariableName=P4_T  SaveFormat=Structure With Time  SampleTime=-1
  wires:
  P/1 -> MATLAB Function/1(u)
  MATLAB Function/1(y) -> Scope24/1, To Workspace/1

== system Cooperative_Quad_09_VelEst_02/Data Bus /Communications for controllers/For matrix Plot4 ==
  A_hat : Inport
  MATLAB Function : MATLAB Function  TreatAsAtomicUnit=on
  Scope24 : Scope
  To Workspace : ToWorkspace  VariableName=A_hat1_T  SaveFormat=Structure With Time  SampleTime=-1
  wires:
  MATLAB Function/1(y) -> Scope24/1, To Workspace/1
  A_hat/1 -> MATLAB Function/1(u)

== system Cooperative_Quad_09_VelEst_02/Data Bus /Communications for controllers/For matrix Plot5 ==
  A_hat : Inport
  MATLAB Function : MATLAB Function  TreatAsAtomicUnit=on
  Scope24 : Scope
  To Workspace : ToWorkspace  VariableName=A_hat2_T  SaveFormat=Structure With Time  SampleTime=-1
  wires:
  A_hat/1 -> MATLAB Function/1(u)
  MATLAB Function/1(y) -> Scope24/1, To Workspace/1

== system Cooperative_Quad_09_VelEst_02/Data Bus /Communications for controllers/For matrix Plot6 ==
  A_hat : Inport
  MATLAB Function : MATLAB Function  TreatAsAtomicUnit=on
  Scope24 : Scope
  To Workspace : ToWorkspace  VariableName=A_hat3_T  SaveFormat=Structure With Time  SampleTime=-1
  wires:
  MATLAB Function/1(y) -> Scope24/1, To Workspace/1
  A_hat/1 -> MATLAB Function/1(u)

== system Cooperative_Quad_09_VelEst_02/Data Bus /Communications for controllers/For matrix Plot7 ==
  A_hat : Inport
  MATLAB Function : MATLAB Function  TreatAsAtomicUnit=on
  Scope24 : Scope
  To Workspace : ToWorkspace  VariableName=A_hat4_T  SaveFormat=Structure With Time  SampleTime=-1
  wires:
  A_hat/1 -> MATLAB Function/1(u)
  MATLAB Function/1(y) -> Scope24/1, To Workspace/1

== system Cooperative_Quad_09_VelEst_02/Data Bus /Reference Trajectory/Differentiator ==
  x_d : Inport
  Integrator : Integrator  InitialCondition=zeros(np,1)
  Integrator1 : Integrator  InitialCondition=zeros(np,1)
  Sliding differentiator : MATLAB Function  TreatAsAtomicUnit=on
  Sliding differentiator1 : MATLAB Function  TreatAsAtomicUnit=on
  Sum : Sum  Inputs=|-+
  Dx_d : Outport
  wires:
  Integrator1/1 -> Sum/2
  Sum/1 -> Sliding differentiator1/1(e), Sliding differentiator/2(e)
  x_d/1 -> Sum/1
  Integrator/1 -> Sliding differentiator/1(u1)
  Sliding differentiator1/1(Du1) -> Integrator/1
  Sliding differentiator/1(u) -> Dx_d/1, Integrator1/1

== system Cooperative_Quad_09_VelEst_02/Data Bus /Reference Trajectory/Differentiator1 ==
  x_d : Inport
  Integrator : Integrator  InitialCondition=zeros(np,1)
  Integrator1 : Integrator  InitialCondition=zeros(np,1)
  Sliding differentiator : MATLAB Function  TreatAsAtomicUnit=on
  Sliding differentiator1 : MATLAB Function  TreatAsAtomicUnit=on
  Sum : Sum  Inputs=|-+
  Dx_d : Outport
  wires:
  Sliding differentiator/1(u) -> Integrator1/1, Dx_d/1
  Sliding differentiator1/1(Du1) -> Integrator/1
  Integrator/1 -> Sliding differentiator/1(u1)
  x_d/1 -> Sum/1
  Sum/1 -> Sliding differentiator/2(e), Sliding differentiator1/1(e)
  Integrator1/1 -> Sum/2

== system Cooperative_Quad_09_VelEst_02/Data Bus /Reference Trajectory/Signal Builder ==
  Demux : Demux  Tag=STV Demux  Outputs=1
  FromWs : FromWorkspace  Tag=STV FromWs  VariableName=tuvar  SampleTime=0
      SigBuilderData=|
      | common.afterFinalStr = 'Extrapolate'
      | common.sampleTime = 0
      | dataSet.timeRange = [0 100]
      | dataSet.name = 'Group 1'
      | sbobj.Groups.Name = 'Group 1'
      | sbobj.Groups.Signals.Name = 'Signal 1'
      | sbobj.Groups.Signals.XData = [0 20 20 50 50 100]
      | sbobj.Groups.Signals.YData = [0 0 2 2 0 0]
      | sbobj.Groups.TimeRange = [0 100]
  Signal 1 : Outport  Tag=STV Outport
  wires:
  Demux/1 -> Signal 1/1
  FromWs/1 -> Demux/1

== system Cooperative_Quad_09_VelEst_02/Data Bus /Reference Trajectory/Subsystem1 ==
  Clock1 : Clock
  Desired Position4 : Constant  Value=0  VectorParams1D=off
  From Workspace : FromWorkspace  VariableName=RECT_X  SampleTime=0
  From Workspace1 : FromWorkspace  VariableName=RECT_Y  SampleTime=0
  From Workspace3 : FromWorkspace  VariableName=RECT_Z  SampleTime=0
  Gain : Gain  Gain=1/2
  Gain1 : Gain  Gain=1/2
  Gain2 : Gain  Gain=1/2
  Scope2 : Scope  NumInputPorts=3
  Switch : Switch  Criteria=u2 > Threshold  Threshold=10
  Xd : Outport
  Yd : Outport  Port=2
  Zd : Outport  Port=3
  wires:
  From Workspace/1 -> Gain/1
  From Workspace1/1 -> Gain1/1
  Clock1/1 -> Switch/2
  Switch/1 -> Zd/1, Scope2/3
  From Workspace3/1 -> Gain2/1
  Desired Position4/1 -> Switch/3
  Gain/1 -> Xd/1, Scope2/1
  Gain1/1 -> Yd/1, Scope2/2
  Gain2/1 -> Switch/1

== system Cooperative_Quad_09_VelEst_02/Data Bus /Reference Trajectory/Subsystem2 ==
  Clock1 : Clock
  Desired Position1 : Constant  Value=3  VectorParams1D=off
  Desired Position2 : Constant  VectorParams1D=off
  Desired Position3 : Constant  Value=-1  VectorParams1D=off
  Desired Position4 : Constant  Value=2  VectorParams1D=off
  Desired Position5 : Constant  Value=0.5  VectorParams1D=off
  Desired Position6 : Constant  Value=-0.5  VectorParams1D=off
  Switch : Switch  Criteria=u2 > Threshold  Threshold=50
  Switch1 : Switch  Criteria=u2 > Threshold  Threshold=50
  Switch2 : Switch  Criteria=u2 > Threshold  Threshold=50
  form_x : Outport
  form_y : Outport  Port=2
  form_z : Outport  Port=3
  wires:
  Desired Position1/1 -> Switch/1
  Switch1/1 -> form_y/1
  Switch2/1 -> form_x/1
  Desired Position4/1 -> Switch/3
  Switch/1 -> form_z/1
  Clock1/1 -> Switch1/2, Switch2/2, Switch/2
  Desired Position2/1 -> Switch1/1
  Desired Position3/1 -> Switch1/3
  Desired Position6/1 -> Switch2/3
  Desired Position5/1 -> Switch2/1

== system Cooperative_Quad_09_VelEst_02/Agent #1/Decenteralized Cooperaive Controller #1/Ali-1/Rotational-1 ==
  x_rd : Inport
  X : Inport  Port=2
  CARE : MATLAB Function  TreatAsAtomicUnit=on
  Differentiator : Subsystem
  Integrator : Integrator  InitialCondition=zeros(n)
  Integrator1 : Integrator  InitialCondition=eye(n)
  Integrator2 : Integrator  InitialCondition=zeros(n,1)
  Integrator3 : Integrator  InitialCondition=zeros(n,1)
  Memory : Memory  InitialCondition=zeros(m,1)
  Sum : Sum  Inputs=|++
  g-Estimator : MATLAB Function  TreatAsAtomicUnit=on
  g-Estimator1 : MATLAB Function  TreatAsAtomicUnit=on
  main : MATLAB Function  TreatAsAtomicUnit=on
  variable change : MATLAB Function  TreatAsAtomicUnit=on
  ur : Outport
  tag scope: A_hat1_R=global, P1_R=global, g_hat1_R=global, u1_R=global
  wires:
  x_rd/1 -> variable change/2(Xd)
  X/1 -> variable change/1(X)
  CARE/1(DP) -> Integrator1/1
  Sum/1 -> main/1(sigma), g-Estimator/1(sigma), g-Estimator1/1(sigma)
  g-Estimator1/1(Da_hat) -> Integrator/1
  variable change/1(x_mod) -> main/7(x), g-Estimator1/2(x)
  Integrator1/1 -> [P1_R], g-Estimator1/3(P), CARE/1(P), g-Estimator/3(P), main/4(P)
  Integrator/1 -> g-Estimator1/4(a_hat), CARE/2(a_hat), [A_hat1_R], main/5(a_hat)
  g-Estimator/1(Dg_hat) -> Integrator2/1
  Differentiator/1(Dx_d) -> main/3(Dy_d)
  main/1(u) -> [u1_R], Memory/1, ur/1
  Integrator3/1 -> main/2(zeta), Sum/1
  variable change/2(xd_mod) -> Differentiator/1(x_d)
  variable change/3(e_mod) -> Sum/2, Integrator3/1
  Memory/1 -> variable change/3(u)
  Integrator2/1 -> g-Estimator/2(g_hat), [g_hat1_R], main/6(g_hat)

== system Cooperative_Quad_09_VelEst_02/Agent #1/Decenteralized Cooperaive Controller #1/Ali-1/Translational-1 ==
  x_td : Inport
  x_t : Inport  Port=2
  A-Estimator : MATLAB Function  TreatAsAtomicUnit=on
  CARE : MATLAB Function  TreatAsAtomicUnit=on
  Differentiator : Subsystem
  Integrator : Integrator  InitialCondition=zeros(n)
  Integrator1 : Integrator  InitialCondition=eye(n)
  Integrator2 : Integrator  InitialCondition=zeros(n,1)
  Integrator3 : Integrator  InitialCondition=zeros(n,1)
  Memory : Memory  InitialCondition=zeros(m,1)
  Sum : Sum  Inputs=|++
  g-Estimator : MATLAB Function  TreatAsAtomicUnit=on
  main : MATLAB Function  TreatAsAtomicUnit=on
  variable change : MATLAB Function  TreatAsAtomicUnit=on
  ut : Outport
  tag scope: A_hat1_T=global, P1_T=global, g_hat1_T=global, u1_T=global
  wires:
  Integrator2/1 -> [g_hat1_T], main/6(g_hat), g-Estimator/2(g_hat)
  Memory/1 -> variable change/3(u)
  variable change/3(e_mod) -> Integrator3/1, Sum/2
  variable change/2(xd_mod) -> Differentiator/1(x_d)
  Integrator3/1 -> Sum/1, main/2(zeta)
  main/1(u) -> ut/1, [u1_T], Memory/1
  Differentiator/1(Dx_d) -> main/3(Dy_d)
  g-Estimator/1(Dg_hat) -> Integrator2/1
  Integrator/1 -> [A_hat1_T], main/5(a_hat), CARE/2(a_hat), A-Estimator/4(a_hat)
  Integrator1/1 -> main/4(P), g-Estimator/3(P), CARE/1(P), [P1_T], A-Estimator/3(P)
  variable change/1(x_mod) -> A-Estimator/2(x), main/7(x)
  A-Estimator/1(Da_hat) -> Integrator/1
  Sum/1 -> A-Estimator/1(sigma), g-Estimator/1(sigma), main/1(sigma)
  CARE/1(DP) -> Integrator1/1
  x_td/1 -> variable change/2(Xd)
  x_t/1 -> variable change/1(X)

== system Cooperative_Quad_09_VelEst_02/Agent #1/Decenteralized Cooperaive Controller #1/Cooperative Observers for X-1/Differentiator2 ==
  Pos_Z : Inport
  Integrator : Integrator
  Integrator1 : Integrator
  Sliding differentiator : MATLAB Function  TreatAsAtomicUnit=on
  Sliding differentiator1 : MATLAB Function  TreatAsAtomicUnit=on
  Sum : Sum  Inputs=|-+
  DPos_Z : Outport
  wires:
  Sliding differentiator/1(u) -> Integrator1/1, DPos_Z/1
  Integrator1/1 -> Sum/2
  Sum/1 -> Sliding differentiator1/1(e), Sliding differentiator/2(e)
  Pos_Z/1 -> Sum/1
  Integrator/1 -> Sliding differentiator/1(u1)
  Sliding differentiator1/1(Du1) -> Integrator/1

== system Cooperative_Quad_09_VelEst_02/Agent #1/Relative estimations-1/Rel_10/Differentiator1 ==
  x_d : Inport
  Constant : Constant  Value=zeros(3,1)
  Gain : Gain
  Integrator : Integrator
  Integrator1 : Integrator
  Sliding differentiator : MATLAB Function  TreatAsAtomicUnit=on
  Sliding differentiator1 : MATLAB Function  TreatAsAtomicUnit=on
  Sum : Sum  Inputs=|-+
  Dx_d : Outport
  wires:
  Sliding differentiator/1(u) -> Integrator1/1, Dx_d/1
  Gain/1 -> Sum/2
  Integrator1/1 -> Gain/1
  Sum/1 -> Sliding differentiator1/1(e), Sliding differentiator/2(e)
  x_d/1 -> Sum/1
  Integrator/1 -> Sliding differentiator/1(u1)
  Sliding differentiator1/1(Du1) -> Integrator/1

== system Cooperative_Quad_09_VelEst_02/Agent #1/Relative estimations-1/Rel_12/Differentiator1 ==
  x_d : Inport
  Constant : Constant  Value=zeros(3,1)
  Gain : Gain
  Integrator : Integrator
  Integrator1 : Integrator
  Sliding differentiator : MATLAB Function  TreatAsAtomicUnit=on
  Sliding differentiator1 : MATLAB Function  TreatAsAtomicUnit=on
  Sum : Sum  Inputs=|-+
  Dx_d : Outport
  wires:
  Sliding differentiator1/1(Du1) -> Integrator/1
  Integrator/1 -> Sliding differentiator/1(u1)
  x_d/1 -> Sum/1
  Sum/1 -> Sliding differentiator/2(e), Sliding differentiator1/1(e)
  Integrator1/1 -> Gain/1
  Gain/1 -> Sum/2
  Sliding differentiator/1(u) -> Dx_d/1, Integrator1/1

== system Cooperative_Quad_09_VelEst_02/Agent #1/Relative estimations-1/Rel_13/Differentiator1 ==
  x_d : Inport
  Constant : Constant  Value=zeros(3,1)
  Gain : Gain
  Integrator : Integrator
  Integrator1 : Integrator
  Sliding differentiator : MATLAB Function  TreatAsAtomicUnit=on
  Sliding differentiator1 : MATLAB Function  TreatAsAtomicUnit=on
  Sum : Sum  Inputs=|-+
  Dx_d : Outport
  wires:
  Sliding differentiator/1(u) -> Integrator1/1, Dx_d/1
  Gain/1 -> Sum/2
  Integrator1/1 -> Gain/1
  Sum/1 -> Sliding differentiator1/1(e), Sliding differentiator/2(e)
  x_d/1 -> Sum/1
  Integrator/1 -> Sliding differentiator/1(u1)
  Sliding differentiator1/1(Du1) -> Integrator/1

== system Cooperative_Quad_09_VelEst_02/Agent #1/Relative estimations-1/Rel_14/Differentiator1 ==
  x_d : Inport
  Constant : Constant  Value=zeros(3,1)
  Gain : Gain
  Integrator : Integrator
  Integrator1 : Integrator
  Sliding differentiator : MATLAB Function  TreatAsAtomicUnit=on
  Sliding differentiator1 : MATLAB Function  TreatAsAtomicUnit=on
  Sum : Sum  Inputs=|-+
  Dx_d : Outport
  wires:
  Sliding differentiator1/1(Du1) -> Integrator/1
  Integrator/1 -> Sliding differentiator/1(u1)
  x_d/1 -> Sum/1
  Sum/1 -> Sliding differentiator/2(e), Sliding differentiator1/1(e)
  Integrator1/1 -> Gain/1
  Gain/1 -> Sum/2
  Sliding differentiator/1(u) -> Dx_d/1, Integrator1/1

== system Cooperative_Quad_09_VelEst_02/Agent #2/Decenteralized Cooperaive Controller #2/Ali-2/Rotational-2 ==
  x_rd : Inport
  X : Inport  Port=2
  CARE : MATLAB Function  TreatAsAtomicUnit=on
  Differentiator : Subsystem
  Integrator : Integrator  InitialCondition=zeros(n)
  Integrator1 : Integrator  InitialCondition=eye(n)
  Integrator2 : Integrator  InitialCondition=zeros(n,1)
  Integrator3 : Integrator  InitialCondition=zeros(n,1)
  Memory : Memory  InitialCondition=zeros(m,1)
  Sum : Sum  Inputs=|++
  g-Estimator : MATLAB Function  TreatAsAtomicUnit=on
  g-Estimator1 : MATLAB Function  TreatAsAtomicUnit=on
  main : MATLAB Function  TreatAsAtomicUnit=on
  variable change : MATLAB Function  TreatAsAtomicUnit=on
  ur : Outport
  tag scope: A_hat2_R=global, P2_R=global, g_hat2_R=global, u2_R=global
  wires:
  Integrator2/1 -> main/6(g_hat), [g_hat2_R], g-Estimator/2(g_hat)
  Memory/1 -> variable change/3(u)
  variable change/3(e_mod) -> Integrator3/1, Sum/2
  variable change/2(xd_mod) -> Differentiator/1(x_d)
  Integrator3/1 -> Sum/1, main/2(zeta)
  main/1(u) -> ur/1, Memory/1, [u2_R]
  Differentiator/1(Dx_d) -> main/3(Dy_d)
  g-Estimator/1(Dg_hat) -> Integrator2/1
  Integrator/1 -> main/5(a_hat), [A_hat2_R], CARE/2(a_hat), g-Estimator1/4(a_hat)
  Integrator1/1 -> main/4(P), g-Estimator/3(P), CARE/1(P), g-Estimator1/3(P), [P2_R]
  variable change/1(x_mod) -> g-Estimator1/2(x), main/7(x)
  g-Estimator1/1(Da_hat) -> Integrator/1
  Sum/1 -> g-Estimator1/1(sigma), g-Estimator/1(sigma), main/1(sigma)
  CARE/1(DP) -> Integrator1/1
  X/1 -> variable change/1(X)
  x_rd/1 -> variable change/2(Xd)

== system Cooperative_Quad_09_VelEst_02/Agent #2/Decenteralized Cooperaive Controller #2/Ali-2/Translational-2 ==
  x_td : Inport
  x_t : Inport  Port=2
  A-Estimator : MATLAB Function  TreatAsAtomicUnit=on
  CARE : MATLAB Function  TreatAsAtomicUnit=on
  Differentiator : Subsystem
  Integrator : Integrator  InitialCondition=zeros(n)
  Integrator1 : Integrator  InitialCondition=eye(n)
  Integrator2 : Integrator  InitialCondition=zeros(n,1)
  Integrator3 : Integrator  InitialCondition=zeros(n,1)
  Memory : Memory  InitialCondition=zeros(m,1)
  Sum : Sum  Inputs=|++
  g-Estimator : MATLAB Function  TreatAsAtomicUnit=on
  main : MATLAB Function  TreatAsAtomicUnit=on
  variable change : MATLAB Function  TreatAsAtomicUnit=on
  ut : Outport
  tag scope: A_hat2_T=global, P2_T=global, g_hat2_T=global, u2_T=global
  wires:
  x_t/1 -> variable change/1(X)
  x_td/1 -> variable change/2(Xd)
  CARE/1(DP) -> Integrator1/1
  Sum/1 -> main/1(sigma), g-Estimator/1(sigma), A-Estimator/1(sigma)
  A-Estimator/1(Da_hat) -> Integrator/1
  variable change/1(x_mod) -> main/7(x), A-Estimator/2(x)
  Integrator1/1 -> A-Estimator/3(P), [P2_T], CARE/1(P), g-Estimator/3(P), main/4(P)
  Integrator/1 -> A-Estimator/4(a_hat), CARE/2(a_hat), main/5(a_hat), [A_hat2_T]
  g-Estimator/1(Dg_hat) -> Integrator2/1
  Differentiator/1(Dx_d) -> main/3(Dy_d)
  main/1(u) -> Memory/1, [u2_T], ut/1
  Integrator3/1 -> main/2(zeta), Sum/1
  variable change/2(xd_mod) -> Differentiator/1(x_d)
  variable change/3(e_mod) -> Sum/2, Integrator3/1
  Memory/1 -> variable change/3(u)
  Integrator2/1 -> g-Estimator/2(g_hat), main/6(g_hat), [g_hat2_T]

== system Cooperative_Quad_09_VelEst_02/Agent #2/Decenteralized Cooperaive Controller #2/Cooperative Observers for X-2/Differentiator2 ==
  Pos_Z : Inport
  Integrator : Integrator
  Integrator1 : Integrator
  Sliding differentiator : MATLAB Function  TreatAsAtomicUnit=on
  Sliding differentiator1 : MATLAB Function  TreatAsAtomicUnit=on
  Sum : Sum  Inputs=|-+
  DPos_Z : Outport
  wires:
  Sliding differentiator1/1(Du1) -> Integrator/1
  Integrator/1 -> Sliding differentiator/1(u1)
  Pos_Z/1 -> Sum/1
  Sum/1 -> Sliding differentiator/2(e), Sliding differentiator1/1(e)
  Integrator1/1 -> Sum/2
  Sliding differentiator/1(u) -> DPos_Z/1, Integrator1/1

== system Cooperative_Quad_09_VelEst_02/Agent #2/Relative estimations-2/Rel_20/Differentiator1 ==
  x_d : Inport
  Constant : Constant  Value=zeros(3,1)
  Gain : Gain
  Integrator : Integrator
  Integrator1 : Integrator
  Sliding differentiator : MATLAB Function  TreatAsAtomicUnit=on
  Sliding differentiator1 : MATLAB Function  TreatAsAtomicUnit=on
  Sum : Sum  Inputs=|-+
  Dx_d : Outport
  wires:
  Sliding differentiator1/1(Du1) -> Integrator/1
  Integrator/1 -> Sliding differentiator/1(u1)
  x_d/1 -> Sum/1
  Sum/1 -> Sliding differentiator/2(e), Sliding differentiator1/1(e)
  Integrator1/1 -> Gain/1
  Gain/1 -> Sum/2
  Sliding differentiator/1(u) -> Dx_d/1, Integrator1/1

== system Cooperative_Quad_09_VelEst_02/Agent #2/Relative estimations-2/Rel_21/Differentiator1 ==
  x_d : Inport
  Constant : Constant  Value=zeros(3,1)
  Gain : Gain
  Integrator : Integrator
  Integrator1 : Integrator
  Sliding differentiator : MATLAB Function  TreatAsAtomicUnit=on
  Sliding differentiator1 : MATLAB Function  TreatAsAtomicUnit=on
  Sum : Sum  Inputs=|-+
  Dx_d : Outport
  wires:
  Sliding differentiator/1(u) -> Integrator1/1, Dx_d/1
  Gain/1 -> Sum/2
  Integrator1/1 -> Gain/1
  Sum/1 -> Sliding differentiator1/1(e), Sliding differentiator/2(e)
  x_d/1 -> Sum/1
  Integrator/1 -> Sliding differentiator/1(u1)
  Sliding differentiator1/1(Du1) -> Integrator/1

== system Cooperative_Quad_09_VelEst_02/Agent #2/Relative estimations-2/Rel_23/Differentiator1 ==
  x_d : Inport
  Constant : Constant  Value=zeros(3,1)
  Gain : Gain
  Integrator : Integrator
  Integrator1 : Integrator
  Sliding differentiator : MATLAB Function  TreatAsAtomicUnit=on
  Sliding differentiator1 : MATLAB Function  TreatAsAtomicUnit=on
  Sum : Sum  Inputs=|-+
  Dx_d : Outport
  wires:
  Sliding differentiator1/1(Du1) -> Integrator/1
  Integrator/1 -> Sliding differentiator/1(u1)
  x_d/1 -> Sum/1
  Sum/1 -> Sliding differentiator/2(e), Sliding differentiator1/1(e)
  Integrator1/1 -> Gain/1
  Gain/1 -> Sum/2
  Sliding differentiator/1(u) -> Dx_d/1, Integrator1/1
